simulink model "BPSK_BladeRF"  (R2023a)
settings: Solver=FixedStepDiscrete  StartTime=0.0  StopTime=inf  RelTol=1e-3
libraries: dspsrcs4 x1
settings Model: Creator=memre  LastModifiedBy=memre
settings DebuggingCC: ParameterPrecisionLossMsg=none

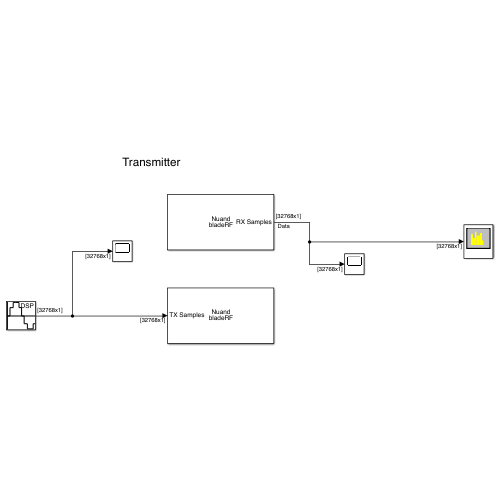
[thumbnail: Simulink's stored preview of the top-level diagram]
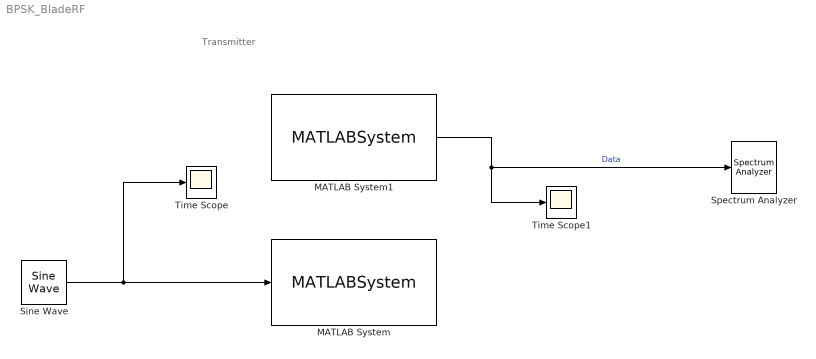
== system BPSK_BladeRF ==
  note: Transmitter
  MATLAB System : MATLABSystem  System=bladeRF_Simulink  device_string=*:instance=1  loopback_mode=None  xb200=off  SimulateUsing=Interpreted execution  enable_rx=off  enable_overrun=off  rx_frequency=sdrqpsktx.BladeRF_Frequency  rx_samplerate=sdrqpsktx.BladeRF_SampleRate  rx_bandwidth=1.5  rx_gain=sdrqpsktx.BladeRF_Gain_Rx  enable_rx_biastee=off  rx_agc=AUTO  rx_num_buffers=sdrqpsktx.BladeRF.stream.n_buffers  rx_num_transfers=sdrqpsktx.BladeRF.stream.n_transfers  rx_buf_size=sdrqpsktx.BladeRF.stream.buffer_size  rx_timeout_ms=sdrqpsktx.BladeRF.stream.timeout  rx_step_size=10000  enable_tx=on  enable_underrun=off  tx_frequency=150e6  tx_samplerate=2.084e6  tx_bandwidth=1.5  tx_gain=sdrqpsktx.BladeRF_Gain_Tx  enable_tx_biastee=off  tx_num_buffers=sdrqpsktx.BladeRF.stream.n_buffers  tx_num_transfers=sdrqpsktx.BladeRF.stream.n_transfers  tx_buf_size=sdrqpsktx.BladeRF.stream.buffer_size  tx_timeout_ms=sdrqpsktx.BladeRF.stream.timeout  tx_step_size=32768  verbosity=Info
      mask Type: bladeRF_Simulink
      mask Display:
      | disp(['Nuand' char(10) 'bladeRF']);
      | port_label('input',1,'TX Samples');
  MATLAB System1 : MATLABSystem  System=bladeRF_Simulink  device_string=*:instance=0  loopback_mode=None  xb200=off  SimulateUsing=Interpreted execution  enable_rx=on  enable_overrun=off  rx_frequency=150e6  rx_samplerate=2.084e6  rx_bandwidth=1.5  rx_gain=30  enable_rx_biastee=off  rx_agc=SLOW  rx_num_buffers=sdrqpsktx.BladeRF.stream.n_buffers  rx_num_transfers=sdrqpsktx.BladeRF.stream.n_transfers  rx_buf_size=sdrqpsktx.BladeRF.stream.buffer_size  rx_timeout_ms=sdrqpsktx.BladeRF.stream.timeout  rx_step_size=32768  enable_tx=off  enable_underrun=off  tx_frequency=sdrqpsktx.BladeRF_Frequency  tx_samplerate=sdrqpsktx.BladeRF_SampleRate  tx_bandwidth=1.5  tx_gain=sdrqpsktx.BladeRF_Gain_Tx  enable_tx_biastee=off  tx_num_buffers=sdrqpsktx.BladeRF.stream.n_buffers  tx_num_transfers=sdrqpsktx.BladeRF.stream.n_transfers  tx_buf_size=sdrqpsktx.BladeRF.stream.buffer_size  tx_timeout_ms=sdrqpsktx.BladeRF.stream.timeout  tx_step_size=10000  verbosity=Info
      mask Type: bladeRF_Simulink
      mask Display:
      | disp(['Nuand' char(10) 'bladeRF']);
      | port_label('output',1,'RX Samples');
  Sine Wave : dspsrcs4/Sine Wave  Amplitude=1  Frequency=50e3  Phase=0  SampleMode=Discrete  OutComplex=Complex  CompMethod=Trigonometric fcn  TableSize=Speed  SampleTime=1/2.084e6  SamplesPerFrame=32768  ResetState=Restart at time zero  OutputFrames=off  dataType=double  wordLen=16  udDataType=sfix(16)  fracBitsMode=Best precision  numFracBits=15  OutDataTypeStr=double  LastOutDataTypeStr=double
  Spectrum Analyzer : SpectrumAnalyzer  WindowPosition=[1136.000000,513.000000,800.000000,500.000000,]  Visible=on  ScopeFrameLocation=window  SpectrumType=Power density  Method=Welch  Span=2084000.0000000002  StartFrequency=-1042000.0000000001  StopFrequency=1042000.0000000001  SpectrumUnits=dBm/Hz  YLimits=[-101.61744769,-22.67661839]  ColorLimits=[-80 20]
  Time Scope : Scope
  Time Scope1 : Scope
  wires:
  Sine Wave/1 -> MATLAB System/1, Time Scope/1
  MATLAB System1/1 -> Spectrum Analyzer/1, Time Scope1/1  "Data"
